simulink model "LLC_ResonanceConverter"  (R2024a)
settings: Solver=daessc  StartTime=0.0  StopTime=2e-3  RelTol=1e-3  AbsTol=1e-3  EnableMultiTasking=on
PreLoadFcn:
  | Vbus_nominal = 450;
  | Vbus_ripple = 10;
  | busRippleFrequency = 100;
  | Vout_nominal = 54;
  | Pout = 100;
  | Cr = 1.2089e-8;
  | Lr = 1.6226e-4;
  | Lm = 2.3e-3;
  | n = 4.3269;
  | transformerCoupling = 0.99;
  | Cout = 3.0237e-5;
  | tdead = 3e-7;
  | fswfinal = [67.287 91.52]*1e3;
  | Vf = 0.6;
  | 
  | switchType = 1;
  | Mode = 0;
InitFcn:
  | clear out;
StopFcn:
  | %ee_addSimlogTimeStamp(bdroot)
  | try
  |     out.SimulationMetadata.TimingInfo
  | catch
  | end
undefined symbols (not defined in the file or in its folder): diff
libraries: ee_lib x12, fl_lib x10, nesl_utility x8, simulink x4, Simscape_lib x2
(part 3 of 3)

== system LLC_ResonanceConverter/Gate Driver/Behavioral Gate Driver/Gate Control Signals/Delayed-on low-side  ==
  u : Inport
  Delayed logic : Logic  AllPortsSameDT=off  OutDataTypeStr=boolean
  One if tdead elapsed : Subsystem  TreatAsAtomicUnit=on
  y : Outport  VectorParamsAs1DForOutWhenUnconnected=off
  wires:
  Delayed logic/1 -> y/1
  One if tdead elapsed/1(y) -> Delayed logic/2
  u/1 -> Delayed logic/1, One if tdead elapsed/Enable

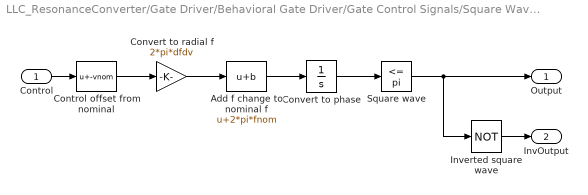
== system LLC_ResonanceConverter/Gate Driver/Behavioral Gate Driver/Gate Control Signals/Square Wave VCO ==
  Control : Inport
  Add f change to nominal f : Bias  Bias=2*pi*fnom  SaturateOnIntegerOverflow=off
  Control offset from nominal : Bias  Bias=-vnom  SaturateOnIntegerOverflow=off
  Convert to phase : Integrator  WrapState=on  WrappedStateUpperValue=2*pi  WrappedStateLowerValue=0
  Convert to radial f : Gain  Gain=2*pi*dfdv
  Inverted square wave : Logic  Operator=NOT  AllPortsSameDT=off  OutDataTypeStr=boolean
  Square wave : simulink/Logic and Bit Operations/Compare To Constant  relop=<=  const=pi  OutDataTypeStr=boolean
  Output : Outport  VectorParamsAs1DForOutWhenUnconnected=off
  InvOutput : Outport  Port=2  VectorParamsAs1DForOutWhenUnconnected=off
  wires:
  Convert to radial f/1 -> Add f change to nominal f/1
  Inverted square wave/1 -> InvOutput/1
  Square wave/1 -> Output/1, Inverted square wave/1
  Convert to phase/1 -> Square wave/1
  Control/1 -> Control offset from nominal/1
  Control offset from nominal/1 -> Convert to radial f/1
  Add f change to nominal f/1 -> Convert to phase/1

== system LLC_ResonanceConverter/Gate Driver/Behavioral Gate Driver/Gate Control Signals/Delayed-on high-side/One if tdead elapsed ==
  Enable : EnablePort  StatesWhenEnabling=reset
  Compare To Constant : simulink/Logic and Bit Operations/Compare To Constant  relop=>  const=tdead  OutDataTypeStr=boolean
  Constant : Constant
  Integrator : Integrator
  y : Outport  VectorParamsAs1DForOutWhenUnconnected=off
  wires:
  Constant/1 -> Integrator/1
  Integrator/1 -> Compare To Constant/1
  Compare To Constant/1 -> y/1

== system LLC_ResonanceConverter/Gate Driver/Behavioral Gate Driver/Gate Control Signals/Delayed-on low-side /One if tdead elapsed ==
  Enable : EnablePort  StatesWhenEnabling=reset
  Compare To Constant : simulink/Logic and Bit Operations/Compare To Constant  relop=>  const=tdead  OutDataTypeStr=boolean
  Constant : Constant
  Integrator : Integrator
  y : Outport  VectorParamsAs1DForOutWhenUnconnected=off
  wires:
  Compare To Constant/1 -> y/1
  Integrator/1 -> Compare To Constant/1
  Constant/1 -> Integrator/1
